simulink model "lead_compensator"  (R2023b)
settings: Solver=VariableStepAuto  StartTime=0.0  StopTime=0.01  RelTol=1e-3
settings Model: Creator=kijun  LastModifiedBy=kijun

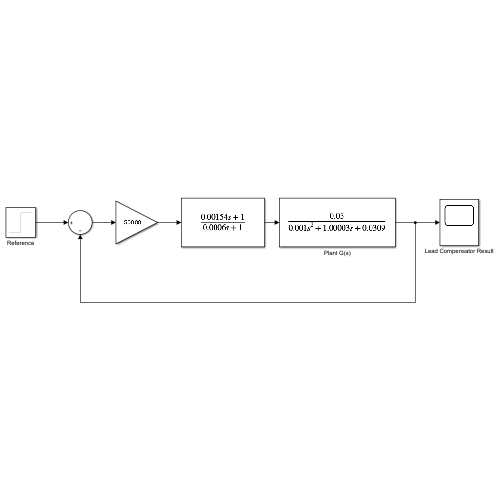
[thumbnail: Simulink's stored preview of the top-level diagram]
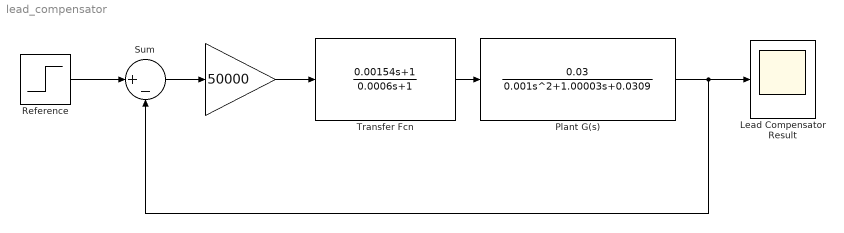
== system lead_compensator ==
  " " : Gain  Gain=50000
  Lead Compensator Result : Scope
  Plant G(s) : TransferFcn  Numerator=[0.03]  Denominator=[0.001 1.00003 0.0309]
  Reference : Step  Time=0  SampleTime=0
  Sum : Sum  Inputs=|+-
  Transfer Fcn : TransferFcn  Numerator=[0.00154 1]  Denominator=[0.0006 1]
  wires:
  Reference/1 -> Sum/1
  Plant G(s)/1 -> Lead Compensator Result/1, Sum/2
  " "/1 -> Transfer Fcn/1
  Transfer Fcn/1 -> Plant G(s)/1
  Sum/1 -> " "/1
